simulink model "generator_model_2026"  (R2016b)
settings: Solver=ode15s  StartTime=0.0  StopTime=0.2  FixedStep=1e-6  MaxStep=1e-5  RelTol=1e-5  EnableMultiTasking=on
InitFcn:
  | Rs=0.42;
  | Ls=0.96e-3;
  | C_phi=92.1952e-3;
  | poles=8;
  | Rload=15;
libraries: powerlib x21
settings Model: Creator=jwjansen  LastModifiedBy=s144150
settings DataIOCC: LimitDataPoints=on  SaveFormat=Array
settings OptimizationCC: ExpressionDepthLimit=2147483647  LifeSpan=inf
settings DebuggingCC: UnderspecifiedInitializationDetection=Classic  MergeDetectMultiDrivingBlocksExec=none  SolverPrmCheckMsg=warning  FcnCallInpInsideContextMsg=warning  UnconnectedInputMsg=none  UnconnectedOutputMsg=none  UnconnectedLineMsg=none  StateNameClashWarn=warning  SFUnexpectedBacktrackingDiag=warning  SFNoUnconditionalDefaultTransitionDiag=warning  SFExecutionAtInitializationDiag=none
settings HardwareCC: ProdBitPerPointer=32  ProdBitPerSizeT=32  ProdBitPerPtrDiffT=32  ProdLargestAtomicFloat=None  ProdIntDivRoundTo=Undefined  ProdEndianess=Unspecified  ProdWordSize=32  ProdHWDeviceType=32-bit Generic
settings ModelReferenceCC: PropagateSignalLabelsOutOfModel=off
settings SFSimCC: SimParseCustomCode=off
settings GRTTargetCC: TargetLangStandard=C89/C90 (ANSI)  GeneratePreprocessorConditionals=Disable all  CombineOutputUpdateFcns=off  GRTInterface=on
settings ConfigComp: CovMetricSettings=dw  CovHtmlReporting=on  CovSaveCumulativeToWorkspaceVar=on  CovSaveSingleToWorkspaceVar=on  CovExternalEMLEnable=off
settings SimscapeCC: SimscapeNormalizeSystem=off

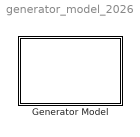
== system generator_model_2026 ==
  " Generator Model " : Subsystem

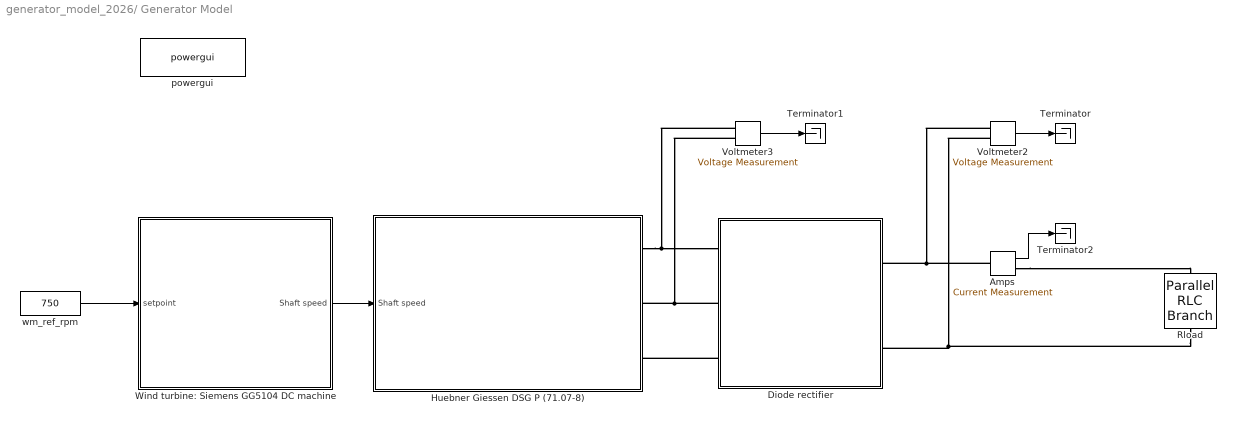
== system generator_model_2026/ Generator Model  ==
  Amps : powerlib/Measurements/Current Measurement  PhasorSimulation=off  OutputType=Complex  PSBequivalent=0
  Diode rectifier : Subsystem
  "Huebner Giessen DSG P (71.07-8) " : Subsystem
  Rload : powerlib/Elements/Parallel RLC Branch  LConnTagsString=a  RConnTagsString=__new0  BranchType=R  Resistance=Rload  Inductance=0.1e-3  SetiL0=off  InitialCurrent=0  Capacitance=1e-3  Setx0=on  InitialVoltage=14  Measurements=Branch voltage and current
  Terminator : Terminator
  Terminator1 : Terminator
  Terminator2 : Terminator
  Voltmeter2 : powerlib/Measurements/Voltage Measurement  PhasorSimulation=off  OutputType=Complex  PSBequivalent=0
  Voltmeter3 : powerlib/Measurements/Voltage Measurement  PhasorSimulation=off  OutputType=Complex  PSBequivalent=0
  "Wind turbine: Siemens GG5104 DC machine " : Subsystem
  powergui : powerlib/powergui  Priority=1  SimulationMode=Continuous  SampleTime=1e-6  frequency=60  Iterations=50  frequencyindice=0  Pbase=100e6  ErrMax=1e-4  UnitsV=kV  UnitsW=MW  buscounter=0  FunctionMessages=off  echomessages=off  EnableUseOfTLC=off  CurrentSourceSwitches=off  DisableSnubberDevices=off  DisableRonSwitches=off  DisableVfSwitches=off  DisplayEquations=off  SolverType=Tustin  Interpol=off  ExternalGateDelay=off  methode=off  Ts=0  x0status=blocks  SPID=off  SwTol=0  HookPort=off  RestoreLinks=warning  ResistiveCurrentMeasurement=off  Frange=[0:2:500]  Ylog=off  Xlog=on  ShowGrid=off  save=off  variable=ZData  structure=0  ZoomFFT=off  StartTime=0.0  cycles=1  DisplayStyle=1  fundamental=60  FreqAxis=off  MaxFrequency=1000  frequencyindicesteady=1  RmsSteady=1  display=off
  wm_ref_rpm : Constant  Value=750
  wires:
  wm_ref_rpm/1 -> "Wind turbine: Siemens GG5104 DC machine "/1(setpoint)
  "Wind turbine: Siemens GG5104 DC machine "/1(Shaft speed) -> "Huebner Giessen DSG P (71.07-8) "/1(Shaft speed)
  Voltmeter2/1 -> Terminator/1
  Voltmeter3/1 -> Terminator1/1
  Amps/1 -> Terminator2/1
  connections:
  "Huebner Giessen DSG P (71.07-8) "/RConn1 -- Voltmeter3/LConn1 -- Diode rectifier/LConn1
  Diode rectifier/LConn2 -- Voltmeter3/LConn2 -- "Huebner Giessen DSG P (71.07-8) "/RConn2
  Diode rectifier/LConn3 -- "Huebner Giessen DSG P (71.07-8) "/RConn3
  Voltmeter2/LConn1 -- Amps/LConn1 -- Diode rectifier/RConn1
  Rload/RConn1 -- Voltmeter2/LConn2 -- Diode rectifier/RConn2
  Amps/RConn1 -- Rload/LConn1

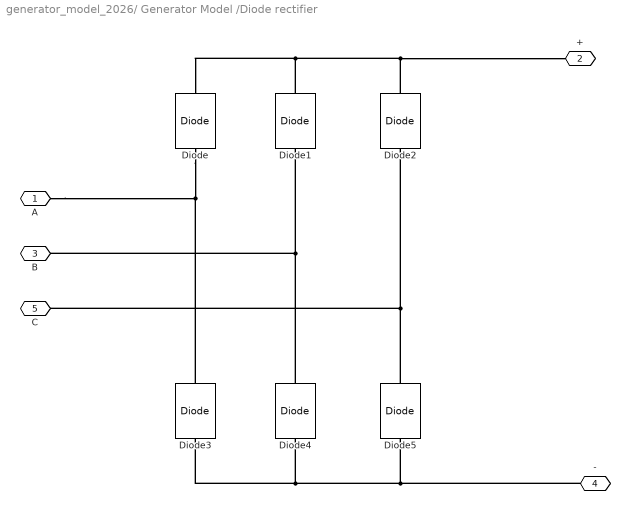
== system generator_model_2026/ Generator Model /Diode rectifier ==
  Diode{,1..5} (6 alike) : powerlib/Power Electronics/Diode  Ron=0.01  Lon=0  Vf=0.85  IC=0  UseSnubber=off  Rs=500  Cs=250e-9  Measurements=off
  A : PMIOPort  Port=1  Side=Left
  + : PMIOPort  Port=2  Side=Right
  B : PMIOPort  Port=3  Side=Left
  - : PMIOPort  Port=4  Side=Right
  C : PMIOPort  Port=5  Side=Left
  connections:
  Diode2/LConn1 -- C/RConn1 -- Diode5/RConn1
  +/RConn1 -- Diode2/RConn1 -- Diode1/RConn1 -- Diode/RConn1
  Diode3/LConn1 -- -/RConn1 -- Diode5/LConn1 -- Diode4/LConn1
  Diode3/RConn1 -- A/RConn1 -- Diode/LConn1
  Diode1/LConn1 -- B/RConn1 -- Diode4/RConn1

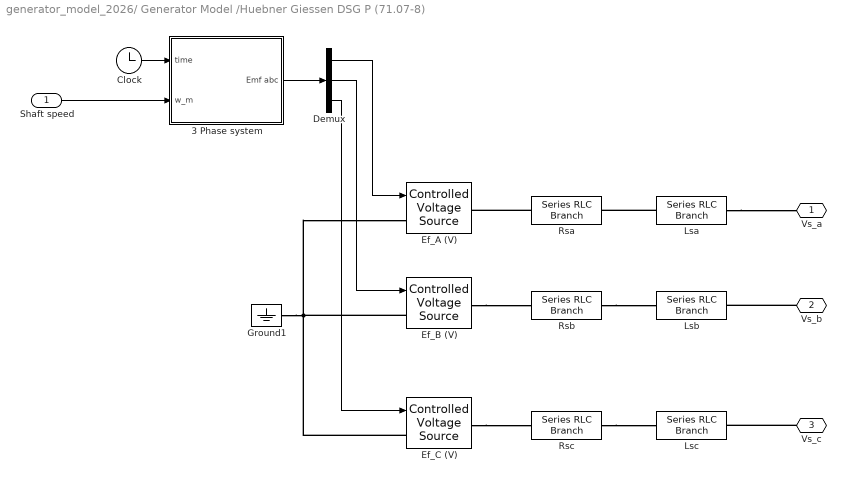
== system generator_model_2026/ Generator Model /Huebner Giessen DSG P (71.07-8)  ==
  Shaft speed : Inport
  "3 Phase system " : Subsystem
  Clock : Clock
  Demux : Demux  Outputs=3
  Ef_A (V) : powerlib/Electrical Sources/Controlled Voltage Source  Initialize=on  Source_Type=AC  Amplitude=0  Phase=0  Frequency=0  Measurements=None
  Ef_B (V) : powerlib/Electrical Sources/Controlled Voltage Source  Initialize=on  Source_Type=AC  Amplitude=0  Phase=0  Frequency=0  Measurements=None
  Ef_C (V) : powerlib/Electrical Sources/Controlled Voltage Source  Initialize=on  Source_Type=AC  Amplitude=0  Phase=0  Frequency=0  Measurements=None
  Ground1 : powerlib/Elements/Ground  LConnTagsString=a
  Lsa : powerlib/Elements/Series RLC Branch  LConnTagsString=__new0  RConnTagsString=__new0  BranchType=L  Resistance=Rs  Inductance=Ls  SetiL0=off  InitialCurrent=0  Capacitance=1e-6  Setx0=off  InitialVoltage=0  Measurements=Branch current
  Lsb : powerlib/Elements/Series RLC Branch  LConnTagsString=__new0  RConnTagsString=__new0  BranchType=L  Resistance=Rs  Inductance=Ls  SetiL0=off  InitialCurrent=0  Capacitance=1e-6  Setx0=off  InitialVoltage=0  Measurements=Branch current
  Lsc : powerlib/Elements/Series RLC Branch  LConnTagsString=__new0  RConnTagsString=__new0  BranchType=L  Resistance=Rs  Inductance=Ls  SetiL0=on  InitialCurrent=0  Capacitance=1e-6  Setx0=off  InitialVoltage=0  Measurements=Branch current
  Rsa : powerlib/Elements/Series RLC Branch  LConnTagsString=__new0  RConnTagsString=__new0  BranchType=R  Resistance=Rs  Inductance=Ls  SetiL0=off  InitialCurrent=0  Capacitance=1e-6  Setx0=off  InitialVoltage=0  Measurements=Branch current
  Rsb : powerlib/Elements/Series RLC Branch  LConnTagsString=__new0  RConnTagsString=__new0  BranchType=R  Resistance=Rs  Inductance=Ls  SetiL0=off  InitialCurrent=0  Capacitance=1e-6  Setx0=off  InitialVoltage=0  Measurements=Branch current
  Rsc : powerlib/Elements/Series RLC Branch  LConnTagsString=__new0  RConnTagsString=__new0  BranchType=R  Resistance=Rs  Inductance=Ls  SetiL0=on  InitialCurrent=0  Capacitance=1e-6  Setx0=off  InitialVoltage=0  Measurements=Branch current
  Vs_a : PMIOPort  Port=1  Side=Right
  Vs_b : PMIOPort  Port=2  Side=Right
  Vs_c : PMIOPort  Port=3  Side=Right
  wires:
  Demux/1 -> Ef_A (V)/1
  Demux/3 -> Ef_C (V)/1
  Demux/2 -> Ef_B (V)/1
  Shaft speed/1 -> "3 Phase system "/2(w_m)
  Clock/1 -> "3 Phase system "/1(time)
  "3 Phase system "/1("Emf abc ") -> Demux/1
  connections:
  Ef_B (V)/RConn1 -- Rsb/LConn1
  Lsa/RConn1 -- Vs_a/RConn1
  Vs_b/RConn1 -- Lsb/RConn1
  Ef_B (V)/LConn1 -- Ground1/LConn1 -- Ef_C (V)/LConn1 -- Ef_A (V)/LConn1
  Vs_c/RConn1 -- Lsc/RConn1
  Lsa/LConn1 -- Rsa/RConn1
  Ef_C (V)/RConn1 -- Rsc/LConn1
  Rsa/LConn1 -- Ef_A (V)/RConn1
  Rsb/RConn1 -- Lsb/LConn1
  Rsc/RConn1 -- Lsc/LConn1

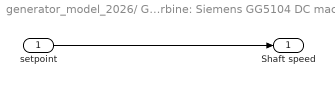
== system generator_model_2026/ Generator Model /Wind turbine: Siemens GG5104 DC machine  ==
  setpoint : Inport
  Shaft speed : Outport
  wires:
  setpoint/1 -> Shaft speed/1

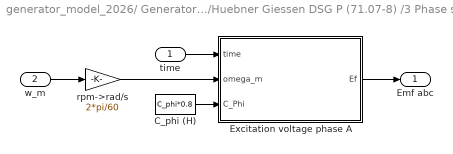
== system generator_model_2026/ Generator Model /Huebner Giessen DSG P (71.07-8) /3 Phase system  ==
  time : Inport
  w_m : Inport  Port=2
  C_phi (H) : Constant  Value=C_phi*0.8  VectorParams1D=off
  Excitation voltage phase A : Subsystem
  rpm->rad/s : Gain  Gain=2*pi/60
  "Emf abc " : Outport
  wires:
  w_m/1 -> rpm->rad/s/1
  C_phi (H)/1 -> Excitation voltage phase A/3(C_Phi)
  time/1 -> Excitation voltage phase A/1(time)
  rpm->rad/s/1 -> Excitation voltage phase A/2(omega_m)
  Excitation voltage phase A/1(Ef) -> "Emf abc "/1

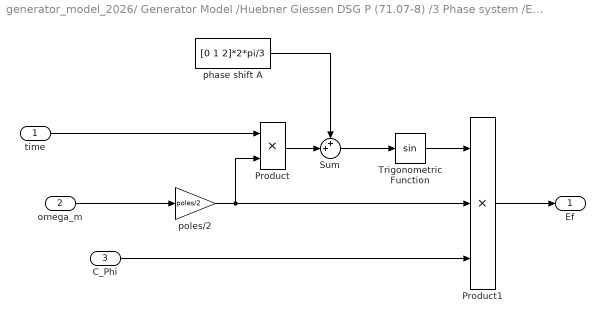
== system generator_model_2026/ Generator Model /Huebner Giessen DSG P (71.07-8) /3 Phase system /Excitation voltage phase A ==
  time : Inport
  omega_m : Inport  Port=2
  C_Phi : Inport  Port=3
  Product : Product  RndMeth=Zero
  Product1 : Product  Inputs=3  RndMeth=Zero
  Sum : Sum  Inputs=++|
  Trigonometric Function : Trigonometry
  phase shift A : Constant  Value=[0 1 2]*2*pi/3
  poles/2 : Gain  Gain=poles/2
  Ef : Outport
  wires:
  poles/2/1 -> Product/2, Product1/2
  Trigonometric Function/1 -> Product1/1
  phase shift A/1 -> Sum/1
  Product/1 -> Sum/2
  Product1/1 -> Ef/1
  C_Phi/1 -> Product1/3
  Sum/1 -> Trigonometric Function/1
  time/1 -> Product/1
  omega_m/1 -> poles/2/1
